simulink model "TransmissionSystem"  (R2026a)
settings: Solver=FixedStepAuto  StopTime=65  FixedStep=0.0005
undefined symbols (not defined in the file): f3ea6d5f
settings Model: DataDictionary=ETRS_data.sldd  VariantConfigurationObject=vConfigData  Creator=macec  LastModifiedBy=burat
settings RTWCC: Toolchain=MinGW64 | gmake (64-bit Windows)

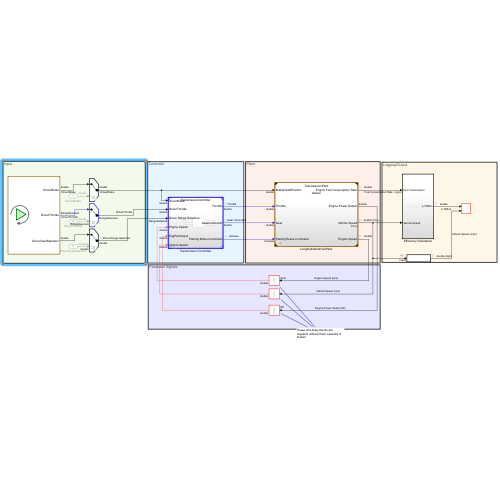
[thumbnail: Simulink's stored preview of the top-level diagram]
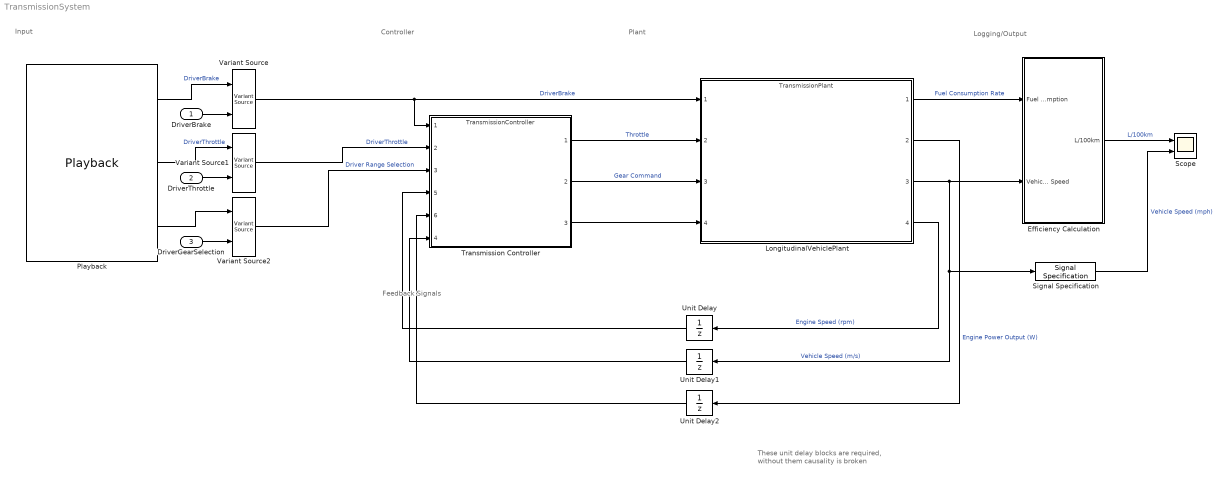
== system TransmissionSystem ==
  note: Logging/Output
  note: These unit delay blocks are required, without them causality is broken
  note: Feedback Signals
  note: Plant
  note: Controller
  note: Input
  DriverBrake : Inport  Interpolate=off
  DriverThrottle : Inport  Port=2  Interpolate=off
  DriverGearSelection : Inport  Port=3  OutDataTypeStr=Enum: RangeSelected  Interpolate=off
  Efficiency Calculation : Subsystem
  LongitudinalVehiclePlant : ModelReference  ModelNameDialog=TransmissionPlant.slx  ModelReferenceVersion=1.91  InputSignalHandling=Zero-order hold
  Playback : Playback  NumPorts=3  PartName=f3ea6d5f-6941-4fcc-8b84-64e5b7c9aa8d  TablePosition=Bottom
  Scope : Scope  NumInputPorts=2
  Signal Specification : SignalSpecification  Unit=mph
  Transmission Controller : ModelReference  ModelNameDialog=TransmissionController  SimulationMode=Normal  ModelReferenceVersion=1.356
      settings: PortSchema="{\"entries\":[{\"content\":{\"sides\":[{\"content\":{\"connectorIds\":[\"In1\",\"In2\",\"In3\",\"In5\",\"In6\",\"In4\"]},\"type\":\"ConnectorPlacement.EquallySpacedRectSide\",\"uuid\":\"61a6d0c1-fe49-48a1-9927-88bd14001373\"},{\"content\":{\"connectorIds\":[\"Out1\",\"Out2\",\"Out3\"],\"side\":\"RIGHT\"},\"type\":\"ConnectorPlacement.EquallySpacedRectSide\",\"uuid\":\"79128b00-5069-4f8a-8a42-773a2caf291f\"},{\"content\":{\"side\":\"TOP\"},\"type\":\"ConnectorPlacement.EquallySpacedRectSide\",\"uuid\":\"32e97420-8a0a-451b-bf14-569133aede3d\"}]},\"type\":\"ConnectorPlacement.EquallySpacedConnector\",\"uuid\":\"34db45d4-e823-4b58-90a9-7f4d94112a06\"}],\"packageUris\":[\"http://schema.mathworks.com/mf0/Connector/R2020b\"],\"version\":\"1.0\"}"
  Unit Delay : UnitDelay  SampleTime=-1
  Unit Delay1 : UnitDelay  SampleTime=-1
  Unit Delay2 : UnitDelay  SampleTime=-1
  Variant Source : VariantSource  VariantControls={V == RunType.Simulate, V == RunType.Test}
  Variant Source1 : VariantSource  VariantControls={V == RunType.Simulate, V == RunType.Test}
  Variant Source2 : VariantSource  VariantControls={V == RunType.Simulate, V == RunType.Test}
  wires:
  Variant Source2/1 -> Transmission Controller/3  "Driver Range Selection"
  Transmission Controller/2 -> LongitudinalVehiclePlant/3  "Gear Command"
  Unit Delay/1 -> Transmission Controller/5
  Unit Delay1/1 -> Transmission Controller/4
  Transmission Controller/1 -> LongitudinalVehiclePlant/2  "Throttle"
  Variant Source/1 -> Transmission Controller/1, LongitudinalVehiclePlant/1  "DriverBrake"
  Variant Source1/1 -> Transmission Controller/2  "DriverThrottle"
  Efficiency Calculation/1(L/100km) -> Scope/1  "L/100km"
  LongitudinalVehiclePlant/4 -> Unit Delay/1  "Engine Speed (rpm)"
  LongitudinalVehiclePlant/3 -> Efficiency Calculation/2(Vehicle Speed), Signal Specification/1, Unit Delay1/1  "Vehicle Speed (m/s)"
  LongitudinalVehiclePlant/1 -> Efficiency Calculation/1(Fuel Consumption)  "Fuel Consumption Rate"
  LongitudinalVehiclePlant/2 -> Unit Delay2/1  "Engine Power Output (W)"
  Playback/1 -> Variant Source/1  "DriverBrake"
  Playback/2 -> Variant Source1/1  "DriverThrottle"
  Playback/3 -> Variant Source2/1
  DriverBrake/1 -> Variant Source/2
  DriverThrottle/1 -> Variant Source1/2
  DriverGearSelection/1 -> Variant Source2/2
  Signal Specification/1 -> Scope/2  "Vehicle Speed (mph)"
  Unit Delay2/1 -> Transmission Controller/6
  Transmission Controller/3 -> LongitudinalVehiclePlant/4

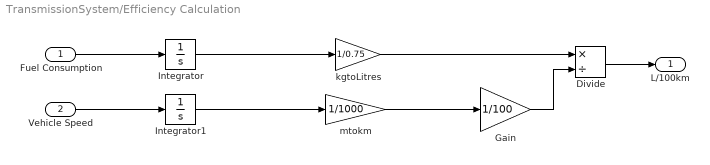
== system TransmissionSystem/Efficiency Calculation ==
  Fuel Consumption : Inport
  Vehicle Speed : Inport  Port=2
  Divide : Product  Inputs=*/
  Gain : Gain  Gain=1/100
  Integrator : Integrator
  Integrator1 : Integrator  InitialCondition=0.0001
  kgtoLitres : Gain  Gain=1/0.75
  mtokm : Gain  Gain=1/1000
  L/100km : Outport
  wires:
  Gain/1 -> Divide/2
  mtokm/1 -> Gain/1
  Vehicle Speed/1 -> Integrator1/1
  Integrator/1 -> kgtoLitres/1
  Integrator1/1 -> mtokm/1
  kgtoLitres/1 -> Divide/1
  Divide/1 -> L/100km/1
  Fuel Consumption/1 -> Integrator/1
